simulink model "HarnessModel_MotorDriveUnit_Inputs"  (R2026a)
settings: Solver=daessc  StopTime=300
PreLoadFcn:
  | MotorDriveUnit.Input_AxleSpeedSwitch_TimePoints = simscape.Value([0, 1], "s");
  | MotorDriveUnit.Input_AxleSpeedSwitch_StepValues = [0 0];
  | 
  | MotorDriveUnit.Input_AxleSpeed_TimePoints = simscape.Value([0, 1, 2], "s");
  | MotorDriveUnit.Input_AxleSpeed_Data = simscape.Value([0, 0, 0], "rpm");
  | 
  | MotorDriveUnit.Input_AxleTorque_TimePoints = simscape.Value([0, 1, 2], "s");
  | MotorDriveUnit.Input_AxleTorque_Data = simscape.Value([-1, -1, -1], "N*m");
  | 
  | MotorDriveUnit.Input_MotorTorqueCommand_TimePoints = simscape.Value([0, 1, 2], "s");
  | MotorDriveUnit.Input_MotorTorqueCommand_Data = simscape.Value([10, 10, 10], "N*m");
  | 
  | MotorDriveUnit.Input_MotorHeatFlow_TimePoints = simscape.Value([0, 1, 2], "s");
  | MotorDriveUnit.Input_MotorHeatFlow_Data = simscape.Value([0, 0, 0], "W");
  | 
  | setupHarness_MotorDriveUnit
settings Model: Creator=isaacito  LastModifiedBy=isaacito
settings SimscapeCC: SimscapeNominalValues="[{\"value\":\"1\",\"unit\":\"A\"},{\"value\":\"1\",\"unit\":\"bar\"},{\"value\":\"1\",\"unit\":\"cm^2\"},{\"value\":\"1\",\"unit\":\"cm^3/s\"},{\"value\":\"1\",\"unit\":\"kJ/kg\"},{\"value\":\"1\",\"unit\":\"kW\"},{\"value\":\"1\",\"unit\":\"l\"},{\"value\":\"1\",\"unit\":\"N\"},{\"value\":\"1\",\"unit\":\"N*m\"},{\"value\":\"1\",\"unit\":\"V\"}]"  SimscapeLogSimulationStatistics=on  SimscapeLogLimitData=off  SimscapeLogDataHistory=5000.0

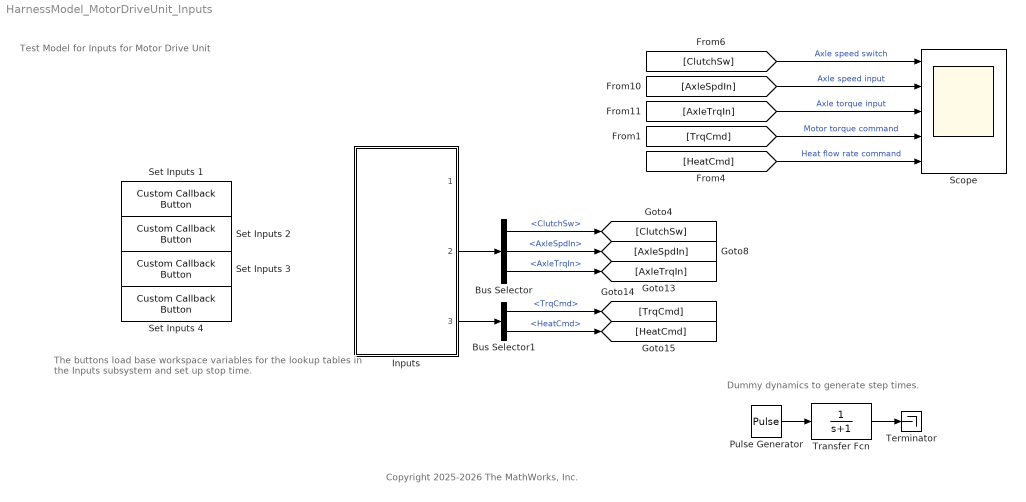
== system HarnessModel_MotorDriveUnit_Inputs ==
  note: The buttons load base workspace variables for the lookup tables in the Inputs subsystem and set up stop time.
  note: Test Model for Inputs for Motor Drive Unit
  note: Copyright 2025-2026 The MathWorks, Inc.
  note: Dummy dynamics to generate step times.
  Bus Selector : BusSelector  OutputSignals=ClutchSw,AxleSpdIn,AxleTrqIn
  Bus Selector1 : BusSelector  OutputSignals=TrqCmd,HeatCmd
  Inputs : Subsystem  ReferencedSubsystem=Inputs_MotorDriveUnit_refsub
  Pulse Generator : DiscretePulseGenerator  PulseType=Time based  PulseWidth=50
  Scope : Scope  NumInputPorts=5
      settings: ActiveDisplayYMinimum=-1  ActiveDisplayYMaximum=1
  Set Inputs 1 : CustomCallbackButton  Configuration="{\"components\":[{\"name\":\"BackgroundImageComponent\",\"settings\":{\"image\":{\"size\":[0,0],\"src\":\"default\",\"srcOrientation\":\"Right\"},\"position\":[0,0,1,1]}},{\"name\":\"ButtonStateComponent\",\"settings\":{\"buttonType\":\"momentary\",\"clickFcn\":\"disp(\\\"Loading inputs: <a href=\\\"\\\"matlab:edit('LoadInputs_MotorDriveUnit_zero')\\\"\\\">LoadInputs_MotorDriveUnit_zero<\\/a>\\\")\\nLoadInputs_MotorDriveUnit_zero\\n\\nset_param(bdroot, StopTime=\\\"10\\\")\\n\\nif get_param(gcs + \\\"\\/Inputs\\\", \\\"ReferencedSubsystem\\\") ~= \\\"Inputs_MotorDriveUnit_refsub\\\"\\n  set_param(gcs + \\\"\\/Inputs\\\", ReferencedSubsystem = \\\"Inputs_MotorDriveUnit_refsub\\\")\\nend\\n\",\"onValue\":1,\"position\":[0,0,1,1],\"pressDelay\":\"500\",\"pressFcn\":\"\",\"repeatInterval\":\"0\",\"states\":[{\"horizontalAlignment\":\"center\",\"image\":{\"position\":[0,0,1,1],\"size\":[1,1],\"src\":\"default\",\"srcOrientation\":\"Right\"},\"label\":{\"color\":[0.01176470588,0.01176470588,0.01176470588,1],\"icon\":{\"size\":[0,0],\"src\":\"default\",\"srcOrientation\":\"Right\"},\"iconOffset\":0,\"iconPlacement\":\"left\",\"opacity\":1,\"show\":true,\"text\":{\"content\":\"Constant\",\"font\":\"Helvetica\"}},\"labelOffset\":[0,0],\"verticalAlignment\":\"middle\"},{\"horizontalAlignment\":\"center\",\"image\":{\"position\":[0,0,1,1],\"size\":[1,1],\"src\":\"default\",\"srcOrientation\":\"Right\"},\"label\":{\"color\":[0.01176470588,0.01176470588,0.01176470588,1],\"icon\":{\"size\":[0,0],\"src\":\"default\",\"srcOrientation\":\"Right\"},\"iconOffset\":0,\"iconPlacement\":\"left\",\"opacity\":1,\"show\":true,\"text\":{\"content\":\"Constant\",\"font\":\"Helvetica\"}},\"labelOffset\":[0,0],\"verticalAlignment\":\"middle\"},{\"horizontalAlignment\":\"center\",\"image\":{\"position\":[0,0,1,1],\"size\":[1,1],\"src\":\"default\",\"srcOrientation\":\"Right\"},\"label\":{\"color\":[0.01176470588,0.01176470588,0.01176470588,1],\"icon\":{\"size\":[0,0],\"src\":\"default\",\"srcOrientation\":\"Right\"},\"iconOffset\":0,\"iconPlacement\":\"left\",\"opacity\":1,\"show\":true,\"text\":{\"content\":\"Constant\",\"font\":\"Helvetica\"}},\"labelOffset\":[0,0],\"verticalAlignment\":\"middle\"},{\"horizontalAlignment\":\"center\",\"image\":{\"position\":[0,0,1,1],\"size\":[1,1],\"src\":\"default\",\"srcOrientation\":\"Right\"},\"label\":{\"color\":[0.01176470588,0.01176470588,0.01176470588,1],\"icon\":{\"size\":[0,0],\"src\":\"default\",\"srcOrientation\":\"Right\"},\"iconOffset\":0,\"iconPlacement\":\"left\",\"opacity\":1,\"show\":true,\"text\":{\"content\":\"Constant\",\"font\":\"Helvetica\"}},\"labelOffset\":[0,0],\"verticalAlignment\":\"middle\"}]}},{\"name\":\"ForegroundImageComponent\",\"settings\":{\"image\":{\"size\":[0,0],\"src\":\"default\",\"srcOrientation\":\"Right\"},\"isForeground\":1,\"position\":[0,0,1,1]}}],\"derived\":{\"blockParameters\":{\"AutoActivate\":true,\"ButtonText\":\"Constant\",\"ButtonType\":\"Momentary\",\"ClickFcn\":\"disp(\\\"Loading inputs: <a href=\\\"\\\"matlab:edit('LoadInputs_MotorDriveUnit_zero')\\\"\\\">LoadInputs_MotorDriveUnit_zero<\\/a>\\\")\\nLoadInputs_MotorDriveUnit_zero\\n\\nset_param(bdroot, StopTime=\\\"10\\\")\\n\\nif get_param(gcs + \\\"\\/Inputs\\\", \\\"ReferencedSubsystem\\\") ~= \\\"Inputs_MotorDriveUnit_refsub\\\"\\n  set_param(gcs + \\\"\\/Inputs\\\", ReferencedSubsystem = \\\"Inputs_MotorDriveUnit_refsub\\\")\\nend\\n\",\"OnValue\":1,\"PressDelay\":\"500\",\"PressFcn\":\"\",\"RepeatInterval\":\"0\",\"fixedAspectRatio\":\"on\"}},\"settings\":{\"BindingType\":\"standalone\",\"autoActivate\":true,\"backgroundColor\":[244,244,244,1],\"backgroundOffset\":0.2,\"backgroundOpacity\":1,\"fixedAspectRatio\":\"on\",\"foregroundColor\":[0.01176470588,0.01176470588,0.01176470588,1],\"migratedFromLegacy\":true,\"useBackgroundColor\":true,\"variant\":\"callback\",\"version\":\"R2025a\"},\"type\":\"Button\"}"  CustomBackgroundColor="{\"color\":[0.9568627451,0.9568627451,0.9568627451],\"show\":true}"
  Set Inputs 2 : CustomCallbackButton  Configuration="{\"components\":[{\"name\":\"BackgroundImageComponent\",\"settings\":{\"image\":{\"size\":[0,0],\"src\":\"default\",\"srcOrientation\":\"Right\"},\"position\":[0,0,1,1]}},{\"name\":\"ButtonStateComponent\",\"settings\":{\"buttonType\":\"momentary\",\"clickFcn\":\"disp(\\\"Loading inputs: <a href=\\\"\\\"matlab:edit('LoadInputs_MotorDriveUnit_Drive')\\\"\\\">LoadInputs_MotorDriveUnit_Drive<\\/a>\\\")\\nLoadInputs_MotorDriveUnit_Drive\\n\\nset_param(bdroot, StopTime=\\\"300\\\")\\n\\nif get_param(gcs + \\\"\\/Inputs\\\", \\\"ReferencedSubsystem\\\") ~= \\\"Inputs_MotorDriveUnit_refsub\\\"\\n  set_param(gcs + \\\"\\/Inputs\\\", ReferencedSubsystem = \\\"Inputs_MotorDriveUnit_refsub\\\")\\nend\\n\",\"onValue\":1,\"position\":[0,0,1,1],\"pressDelay\":\"500\",\"pressFcn\":\"\",\"repeatInterval\":\"0\",\"states\":[{\"horizontalAlignment\":\"center\",\"image\":{\"position\":[0,0,1,1],\"size\":[1,1],\"src\":\"default\",\"srcOrientation\":\"Right\"},\"label\":{\"color\":[0.01176470588,0.01176470588,0.01176470588,1],\"icon\":{\"size\":[0,0],\"src\":\"default\",\"srcOrientation\":\"Right\"},\"iconOffset\":0,\"iconPlacement\":\"left\",\"opacity\":1,\"show\":true,\"text\":{\"content\":\"Drive\",\"font\":\"Helvetica\"}},\"labelOffset\":[0,0],\"verticalAlignment\":\"middle\"},{\"horizontalAlignment\":\"center\",\"image\":{\"position\":[0,0,1,1],\"size\":[1,1],\"src\":\"default\",\"srcOrientation\":\"Right\"},\"label\":{\"color\":[0.01176470588,0.01176470588,0.01176470588,1],\"icon\":{\"size\":[0,0],\"src\":\"default\",\"srcOrientation\":\"Right\"},\"iconOffset\":0,\"iconPlacement\":\"left\",\"opacity\":1,\"show\":true,\"text\":{\"content\":\"Drive\",\"font\":\"Helvetica\"}},\"labelOffset\":[0,0],\"verticalAlignment\":\"middle\"},{\"horizontalAlignment\":\"center\",\"image\":{\"position\":[0,0,1,1],\"size\":[1,1],\"src\":\"default\",\"srcOrientation\":\"Right\"},\"label\":{\"color\":[0.01176470588,0.01176470588,0.01176470588,1],\"icon\":{\"size\":[0,0],\"src\":\"default\",\"srcOrientation\":\"Right\"},\"iconOffset\":0,\"iconPlacement\":\"left\",\"opacity\":1,\"show\":true,\"text\":{\"content\":\"Drive\",\"font\":\"Helvetica\"}},\"labelOffset\":[0,0],\"verticalAlignment\":\"middle\"},{\"horizontalAlignment\":\"center\",\"image\":{\"position\":[0,0,1,1],\"size\":[1,1],\"src\":\"default\",\"srcOrientation\":\"Right\"},\"label\":{\"color\":[0.01176470588,0.01176470588,0.01176470588,1],\"icon\":{\"size\":[0,0],\"src\":\"default\",\"srcOrientation\":\"Right\"},\"iconOffset\":0,\"iconPlacement\":\"left\",\"opacity\":1,\"show\":true,\"text\":{\"content\":\"Drive\",\"font\":\"Helvetica\"}},\"labelOffset\":[0,0],\"verticalAlignment\":\"middle\"}]}},{\"name\":\"ForegroundImageComponent\",\"settings\":{\"image\":{\"size\":[0,0],\"src\":\"default\",\"srcOrientation\":\"Right\"},\"isForeground\":1,\"position\":[0,0,1,1]}}],\"derived\":{\"blockParameters\":{\"AutoActivate\":true,\"ButtonText\":\"Drive\",\"ButtonType\":\"Momentary\",\"ClickFcn\":\"disp(\\\"Loading inputs: <a href=\\\"\\\"matlab:edit('LoadInputs_MotorDriveUnit_Drive')\\\"\\\">LoadInputs_MotorDriveUnit_Drive<\\/a>\\\")\\nLoadInputs_MotorDriveUnit_Drive\\n\\nset_param(bdroot, StopTime=\\\"300\\\")\\n\\nif get_param(gcs + \\\"\\/Inputs\\\", \\\"ReferencedSubsystem\\\") ~= \\\"Inputs_MotorDriveUnit_refsub\\\"\\n  set_param(gcs + \\\"\\/Inputs\\\", ReferencedSubsystem = \\\"Inputs_MotorDriveUnit_refsub\\\")\\nend\\n\",\"OnValue\":1,\"PressDelay\":\"500\",\"PressFcn\":\"\",\"RepeatInterval\":\"0\",\"fixedAspectRatio\":\"on\"}},\"settings\":{\"BindingType\":\"standalone\",\"autoActivate\":true,\"backgroundColor\":[244,244,244,1],\"backgroundOffset\":0.2,\"backgroundOpacity\":1,\"fixedAspectRatio\":\"on\",\"foregroundColor\":[0.01176470588,0.01176470588,0.01176470588,1],\"migratedFromLegacy\":true,\"useBackgroundColor\":true,\"variant\":\"callback\",\"version\":\"R2025a\"},\"type\":\"Button\"}"  CustomBackgroundColor="{\"color\":[0.9568627451,0.9568627451,0.9568627451],\"show\":true}"
  Set Inputs 3 : CustomCallbackButton  Configuration="{\"components\":[{\"name\":\"BackgroundImageComponent\",\"settings\":{\"image\":{\"size\":[0,0],\"src\":\"default\",\"srcOrientation\":\"Right\"},\"position\":[0,0,1,1]}},{\"name\":\"ButtonStateComponent\",\"settings\":{\"buttonType\":\"momentary\",\"clickFcn\":\"disp(\\\"Loading inputs: <a href=\\\"\\\"matlab:edit('LoadInputs_MotorDriveUnit_Regen')\\\"\\\">LoadInputs_MotorDriveUnit_Regen<\\/a>\\\")\\nLoadInputs_MotorDriveUnit_Regen\\n\\nset_param(bdroot, StopTime=\\\"400\\\")\\n\\nif get_param(gcs + \\\"\\/Inputs\\\", \\\"ReferencedSubsystem\\\") ~= \\\"Inputs_MotorDriveUnit_refsub\\\"\\n  set_param(gcs + \\\"\\/Inputs\\\", ReferencedSubsystem = \\\"Inputs_MotorDriveUnit_refsub\\\")\\nend\\n\",\"onValue\":1,\"position\":[0,0,1,1],\"pressDelay\":\"500\",\"pressFcn\":\"\",\"repeatInterval\":\"0\",\"states\":[{\"horizontalAlignment\":\"center\",\"image\":{\"position\":[0,0,1,1],\"size\":[1,1],\"src\":\"default\",\"srcOrientation\":\"Right\"},\"label\":{\"color\":[0.01176470588,0.01176470588,0.01176470588,1],\"icon\":{\"size\":[0,0],\"src\":\"default\",\"srcOrientation\":\"Right\"},\"iconOffset\":0,\"iconPlacement\":\"left\",\"opacity\":1,\"show\":true,\"text\":{\"content\":\"Regen Brake\",\"font\":\"Helvetica\"}},\"labelOffset\":[0,0],\"verticalAlignment\":\"middle\"},{\"horizontalAlignment\":\"center\",\"image\":{\"position\":[0,0,1,1],\"size\":[1,1],\"src\":\"default\",\"srcOrientation\":\"Right\"},\"label\":{\"color\":[0.01176470588,0.01176470588,0.01176470588,1],\"icon\":{\"size\":[0,0],\"src\":\"default\",\"srcOrientation\":\"Right\"},\"iconOffset\":0,\"iconPlacement\":\"left\",\"opacity\":1,\"show\":true,\"text\":{\"content\":\"Regen Brake\",\"font\":\"Helvetica\"}},\"labelOffset\":[0,0],\"verticalAlignment\":\"middle\"},{\"horizontalAlignment\":\"center\",\"image\":{\"position\":[0,0,1,1],\"size\":[1,1],\"src\":\"default\",\"srcOrientation\":\"Right\"},\"label\":{\"color\":[0.01176470588,0.01176470588,0.01176470588,1],\"icon\":{\"size\":[0,0],\"src\":\"default\",\"srcOrientation\":\"Right\"},\"iconOffset\":0,\"iconPlacement\":\"left\",\"opacity\":1,\"show\":true,\"text\":{\"content\":\"Regen Brake\",\"font\":\"Helvetica\"}},\"labelOffset\":[0,0],\"verticalAlignment\":\"middle\"},{\"horizontalAlignment\":\"center\",\"image\":{\"position\":[0,0,1,1],\"size\":[1,1],\"src\":\"default\",\"srcOrientation\":\"Right\"},\"label\":{\"color\":[0.01176470588,0.01176470588,0.01176470588,1],\"icon\":{\"size\":[0,0],\"src\":\"default\",\"srcOrientation\":\"Right\"},\"iconOffset\":0,\"iconPlacement\":\"left\",\"opacity\":1,\"show\":true,\"text\":{\"content\":\"Regen Brake\",\"font\":\"Helvetica\"}},\"labelOffset\":[0,0],\"verticalAlignment\":\"middle\"}]}},{\"name\":\"ForegroundImageComponent\",\"settings\":{\"image\":{\"size\":[0,0],\"src\":\"default\",\"srcOrientation\":\"Right\"},\"isForeground\":1,\"position\":[0,0,1,1]}}],\"derived\":{\"blockParameters\":{\"AutoActivate\":true,\"ButtonText\":\"Regen Brake\",\"ButtonType\":\"Momentary\",\"ClickFcn\":\"disp(\\\"Loading inputs: <a href=\\\"\\\"matlab:edit('LoadInputs_MotorDriveUnit_Regen')\\\"\\\">LoadInputs_MotorDriveUnit_Regen<\\/a>\\\")\\nLoadInputs_MotorDriveUnit_Regen\\n\\nset_param(bdroot, StopTime=\\\"400\\\")\\n\\nif get_param(gcs + \\\"\\/Inputs\\\", \\\"ReferencedSubsystem\\\") ~= \\\"Inputs_MotorDriveUnit_refsub\\\"\\n  set_param(gcs + \\\"\\/Inputs\\\", ReferencedSubsystem = \\\"Inputs_MotorDriveUnit_refsub\\\")\\nend\\n\",\"OnValue\":1,\"PressDelay\":\"500\",\"PressFcn\":\"\",\"RepeatInterval\":\"0\",\"fixedAspectRatio\":\"on\"}},\"settings\":{\"BindingType\":\"standalone\",\"autoActivate\":true,\"backgroundColor\":[244,244,244,1],\"backgroundOffset\":0.2,\"backgroundOpacity\":1,\"fixedAspectRatio\":\"on\",\"foregroundColor\":[0.01176470588,0.01176470588,0.01176470588,1],\"migratedFromLegacy\":true,\"useBackgroundColor\":true,\"variant\":\"callback\",\"version\":\"R2025a\"},\"type\":\"Button\"}"  CustomBackgroundColor="{\"color\":[0.9568627451,0.9568627451,0.9568627451],\"show\":true}"
  Set Inputs 4 : CustomCallbackButton  Configuration="{\"components\":[{\"name\":\"BackgroundImageComponent\",\"settings\":{\"image\":{\"size\":[0,0],\"src\":\"default\",\"srcOrientation\":\"Right\"},\"position\":[0,0,1,1]}},{\"name\":\"ButtonStateComponent\",\"settings\":{\"buttonType\":\"momentary\",\"clickFcn\":\"disp(\\\"Loading inputs: <a href=\\\"\\\"matlab:edit('LoadInputs_MotorDriveUnit_Random')\\\"\\\">LoadInputs_MotorDriveUnit_Random<\\/a>\\\")\\nLoadInputs_MotorDriveUnit_Random\\n\\nset_param(bdroot, StopTime=\\\"400\\\")\\n\\nif get_param(gcs + \\\"\\/Inputs\\\", \\\"ReferencedSubsystem\\\") ~= \\\"Inputs_MotorDriveUnit_refsub\\\"\\n  set_param(gcs + \\\"\\/Inputs\\\", ReferencedSubsystem = \\\"Inputs_MotorDriveUnit_refsub\\\")\\nend\\n\",\"onValue\":1,\"position\":[0,0,1,1],\"pressDelay\":\"500\",\"pressFcn\":\"\",\"repeatInterval\":\"0\",\"states\":[{\"horizontalAlignment\":\"center\",\"image\":{\"position\":[0,0,1,1],\"size\":[1,1],\"src\":\"default\",\"srcOrientation\":\"Right\"},\"label\":{\"color\":[0.01176470588,0.01176470588,0.01176470588,1],\"icon\":{\"size\":[0,0],\"src\":\"default\",\"srcOrientation\":\"Right\"},\"iconOffset\":0,\"iconPlacement\":\"left\",\"opacity\":1,\"show\":true,\"text\":{\"content\":\"Random\",\"font\":\"Helvetica\"}},\"labelOffset\":[0,0],\"verticalAlignment\":\"middle\"},{\"horizontalAlignment\":\"center\",\"image\":{\"position\":[0,0,1,1],\"size\":[1,1],\"src\":\"default\",\"srcOrientation\":\"Right\"},\"label\":{\"color\":[0.01176470588,0.01176470588,0.01176470588,1],\"icon\":{\"size\":[0,0],\"src\":\"default\",\"srcOrientation\":\"Right\"},\"iconOffset\":0,\"iconPlacement\":\"left\",\"opacity\":1,\"show\":true,\"text\":{\"content\":\"Random\",\"font\":\"Helvetica\"}},\"labelOffset\":[0,0],\"verticalAlignment\":\"middle\"},{\"horizontalAlignment\":\"center\",\"image\":{\"position\":[0,0,1,1],\"size\":[1,1],\"src\":\"default\",\"srcOrientation\":\"Right\"},\"label\":{\"color\":[0.01176470588,0.01176470588,0.01176470588,1],\"icon\":{\"size\":[0,0],\"src\":\"default\",\"srcOrientation\":\"Right\"},\"iconOffset\":0,\"iconPlacement\":\"left\",\"opacity\":1,\"show\":true,\"text\":{\"content\":\"Random\",\"font\":\"Helvetica\"}},\"labelOffset\":[0,0],\"verticalAlignment\":\"middle\"},{\"horizontalAlignment\":\"center\",\"image\":{\"position\":[0,0,1,1],\"size\":[1,1],\"src\":\"default\",\"srcOrientation\":\"Right\"},\"label\":{\"color\":[0.01176470588,0.01176470588,0.01176470588,1],\"icon\":{\"size\":[0,0],\"src\":\"default\",\"srcOrientation\":\"Right\"},\"iconOffset\":0,\"iconPlacement\":\"left\",\"opacity\":1,\"show\":true,\"text\":{\"content\":\"Random\",\"font\":\"Helvetica\"}},\"labelOffset\":[0,0],\"verticalAlignment\":\"middle\"}]}},{\"name\":\"ForegroundImageComponent\",\"settings\":{\"image\":{\"size\":[0,0],\"src\":\"default\",\"srcOrientation\":\"Right\"},\"isForeground\":1,\"position\":[0,0,1,1]}}],\"derived\":{\"blockParameters\":{\"AutoActivate\":true,\"ButtonText\":\"Random\",\"ButtonType\":\"Momentary\",\"ClickFcn\":\"disp(\\\"Loading inputs: <a href=\\\"\\\"matlab:edit('LoadInputs_MotorDriveUnit_Random')\\\"\\\">LoadInputs_MotorDriveUnit_Random<\\/a>\\\")\\nLoadInputs_MotorDriveUnit_Random\\n\\nset_param(bdroot, StopTime=\\\"400\\\")\\n\\nif get_param(gcs + \\\"\\/Inputs\\\", \\\"ReferencedSubsystem\\\") ~= \\\"Inputs_MotorDriveUnit_refsub\\\"\\n  set_param(gcs + \\\"\\/Inputs\\\", ReferencedSubsystem = \\\"Inputs_MotorDriveUnit_refsub\\\")\\nend\\n\",\"OnValue\":1,\"PressDelay\":\"500\",\"PressFcn\":\"\",\"RepeatInterval\":\"0\",\"fixedAspectRatio\":\"on\"}},\"settings\":{\"BindingType\":\"standalone\",\"autoActivate\":true,\"backgroundColor\":[244,244,244,1],\"backgroundOffset\":0.2,\"backgroundOpacity\":1,\"fixedAspectRatio\":\"on\",\"foregroundColor\":[0.01176470588,0.01176470588,0.01176470588,1],\"migratedFromLegacy\":true,\"useBackgroundColor\":true,\"variant\":\"callback\",\"version\":\"R2025a\"},\"type\":\"Button\"}"  CustomBackgroundColor="{\"color\":[0.9568627451,0.9568627451,0.9568627451],\"show\":true}"
  Terminator : Terminator
  Transfer Fcn : TransferFcn  Denominator=[1 1]
  wires:
  Inputs/2 -> Bus Selector/1
  Bus Selector/2 -> [AxleSpdIn]  "<AxleSpdIn>"
  Bus Selector/3 -> [AxleTrqIn]  "<AxleTrqIn>"
  Bus Selector/1 -> [ClutchSw]  "<ClutchSw>"
  Inputs/3 -> Bus Selector1/1
  Bus Selector1/1 -> [TrqCmd]  "<TrqCmd>"
  Bus Selector1/2 -> [HeatCmd]  "<HeatCmd>"
  [ClutchSw] -> Scope/1  "Axle speed switch"
  [AxleSpdIn] -> Scope/2  "Axle speed input"
  [AxleTrqIn] -> Scope/3  "Axle torque input"
  [TrqCmd] -> Scope/4  "Motor torque command"
  [HeatCmd] -> Scope/5  "Heat flow rate command"
  Pulse Generator/1 -> Transfer Fcn/1
  Transfer Fcn/1 -> Terminator/1
